simulink model "chap5_1sim"  (Simulink 7.7)
settings: Solver=ode45  StartTime=0.0  StopTime=5.0  FixedStep=0.001  RelTol=1e-3
PreLoadFcn:
  | i=k;
values from neighbouring files (symbols this model uses):
  k = k'    [chap5_1main.m]    (also in chap5_2main.m; chap5_3main.m; chap5_4main.m; chap5_5main.m)
settings Model: Creator=ljk  LastModifiedBy=ljk
settings DataIOCC: MaxDataPoints=10000  SignalLoggingName=sigsOut
settings DebuggingCC: SaveWithParameterizedLinksMsg=none  SignalResolutionControl=TryResolveAllWithWarning  SolverPrmCheckMsg=none  MultiTaskDSMMsg=warning  MultiTaskCondExecSysMsg=none  StrictBusMsg=None
settings HardwareCC: TargetUnknown=on
settings RTWCC: IncludeERTFirstTime=on

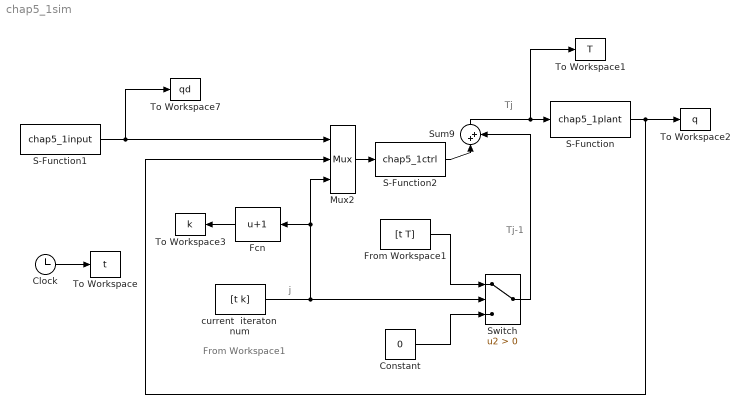
== system chap5_1sim ==
  note: Tj
  note: Tj-1
  note: j
  note: From
      | Workspace1
  Clock : Clock
      settings: Decimation=10
  Constant : Constant  Value=0
  Fcn : Fcn  Expr=u+1
  From Workspace1 : FromWorkspace  VariableName=[t T]  SampleTime=0
  Mux2 : Mux  Inputs=3
  S-Function : S-Function  FunctionName=chap5_1plant  EnableBusSupport=off
  S-Function1 : S-Function  FunctionName=chap5_1input  EnableBusSupport=off
  S-Function2 : S-Function  FunctionName=chap5_1ctrl  EnableBusSupport=off
  Sum9 : Sum  Inputs=|++  SaturateOnIntegerOverflow=on
  Switch : Switch  Criteria=u2 > Threshold  SaturateOnIntegerOverflow=on
  To Workspace : ToWorkspace  VariableName=t  SampleTime=-1  SaveFormat=Array
  To Workspace1 : ToWorkspace  VariableName=T  SampleTime=-1  SaveFormat=Array
  To Workspace2 : ToWorkspace  VariableName=q  SampleTime=-1  SaveFormat=Array
  To Workspace3 : ToWorkspace  VariableName=k  SampleTime=-1  SaveFormat=Array
  To Workspace7 : ToWorkspace  VariableName=qd  SampleTime=-1  SaveFormat=Array
  current  iteraton  num : FromWorkspace  VariableName=[t k]  SampleTime=0
  wires:
  S-Function/1 -> To Workspace2/1, Mux2/2
  Clock/1 -> To Workspace/1
  S-Function1/1 -> To Workspace7/1, Mux2/1
  S-Function2/1 -> Sum9/1
  Sum9/1 -> S-Function/1, To Workspace1/1
  Switch/1 -> Sum9/2
  Constant/1 -> Switch/3
  Mux2/1 -> S-Function2/1
  From Workspace1/1 -> Switch/1
  current  iteraton  num/1 -> Switch/2, Fcn/1, Mux2/3
  Fcn/1 -> To Workspace3/1
